simulink model "FM_Modulation_Demodulation_01"  (R2021b)
settings: Solver=VariableStepAuto  StartTime=0.0  StopTime=50  RelTol=1e-3
undefined symbols (not defined in the file): DiscIntNeverNeededParam
libraries: dsparch4 x1, commsynccomp2 x1, commanapbnd3 x1
settings Model: Creator=Rajeev Ranjan  LastModifiedBy=Rajeev Ranjan

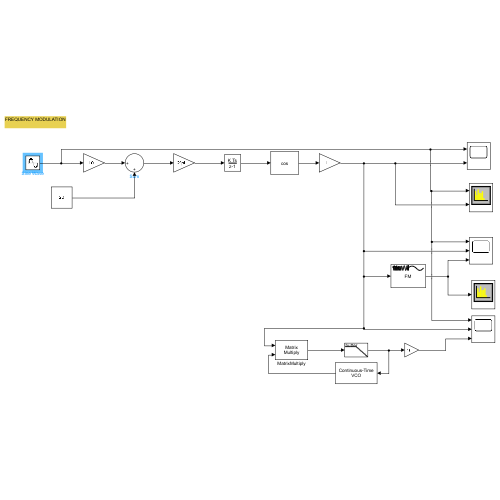
[thumbnail: Simulink's stored preview of the top-level diagram]
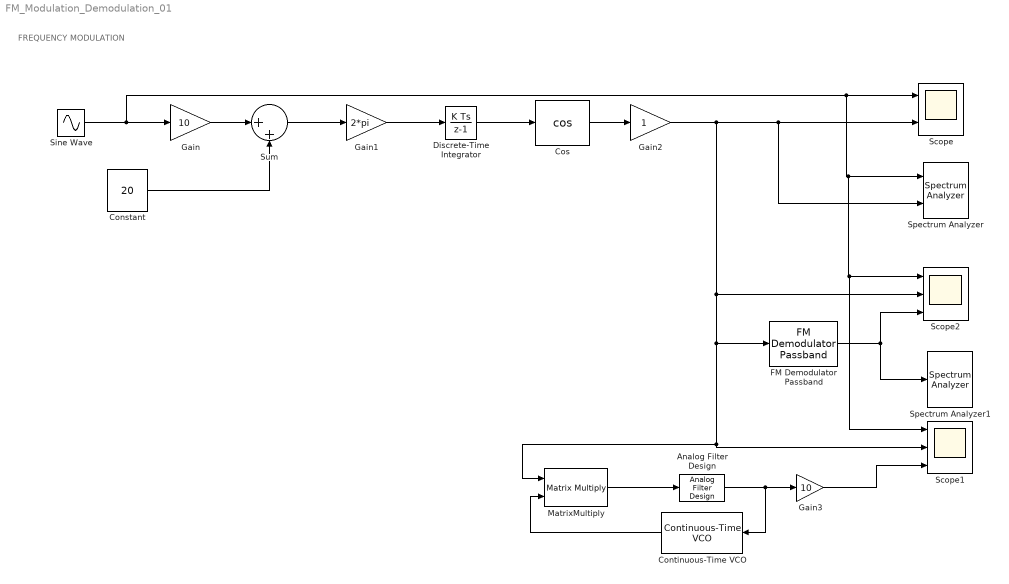
== system FM_Modulation_Demodulation_01 ==
  note: FREQUENCY MODULATION
  Analog Filter Design : dsparch4/Analog Filter Design  method=Butterworth  filttype=Lowpass  N=10  Wlo=2  Whi=80  Rp=2  Rs=40
  Constant : Constant  Value=20
  Continuous-Time VCO : commsynccomp2/Continuous-Time VCO  Ac=1  Fc=20  Kc=10/(2*pi)  Ph=pi/2
      settings: SourceProductBaseCode=CM
  Cos : Trigonometry  Operator=cos
  Discrete-Time Integrator : DiscreteIntegrator  SampleTime=-1  ICPrevOutput=DiscIntNeverNeededParam  ICPrevScaledInput=DiscIntNeverNeededParam
  FM Demodulator Passband : commanapbnd3/FM Demodulator Passband  Fc=20  Ph=0  Kc=10  Ho=200
      settings: SourceProductBaseCode=CM
  Gain : Gain  Gain=10
  Gain1 : Gain  Gain=2*pi
  Gain2 : Gain
  Gain3 : Gain  Gain=10
  MatrixMultiply : Product  Multiplication=Matrix(*)
  Scope : Scope  NumInputPorts=2
  Scope1 : Scope  NumInputPorts=3
  Scope2 : Scope  NumInputPorts=3
  Sine Wave : Sin  Frequency=2  SampleTime=1/1000
  Spectrum Analyzer : SpectrumAnalyzer  NumInputPorts=2
  Spectrum Analyzer1 : SpectrumAnalyzer
  Sum : Sum  Inputs=|++
  wires:
  Gain/1 -> Sum/1
  Constant/1 -> Sum/2
  Sine Wave/1 -> Scope1/1, Scope2/1, Spectrum Analyzer/1, Scope/1, Gain/1
  Sum/1 -> Gain1/1
  Gain1/1 -> Discrete-Time Integrator/1
  Discrete-Time Integrator/1 -> Cos/1
  Cos/1 -> Gain2/1
  Gain2/1 -> Scope2/2, MatrixMultiply/1, Scope1/2, FM Demodulator Passband/1, Spectrum Analyzer/2, Scope/2
  FM Demodulator Passband/1 -> Spectrum Analyzer1/1, Scope2/3
  MatrixMultiply/1 -> Analog Filter Design/1
  Analog Filter Design/1 -> Continuous-Time VCO/1, Gain3/1
  Gain3/1 -> Scope1/3
  Continuous-Time VCO/1 -> MatrixMultiply/2
